simulink model "SendToUdpServer"  (R2018a)
settings: Solver=FixedStepAuto  StartTime=0.0  StopTime=inf  RelTol=1e-3  EnableMultiTasking=on
libraries: arduinowifilib x1
settings Model: SimulationMode=external  ExtModeTrigDuration=2  Creator=Gerard  LastModifiedBy=gaharkem
settings OptimizationCC: EnhancedBackFolding=on  PassReuseOutputArgsThreshold=0  MaxStackSize=64  OptimizeBlockOrder=speed  DifferentSizesBufferReuse=on  OptimizationCustomize=off
settings DebuggingCC: ParameterTunabilityLossMsg=error  LibraryContextMissingDiagnostic=warning
settings HardwareCC: ProdBitPerPointer=32  ProdBitPerSizeT=32  ProdBitPerPtrDiffT=32  ProdLargestAtomicInteger=Long  ProdLargestAtomicFloat=Double  ProdWordSize=32  ProdHWDeviceType=ARM Compatible->ARM Cortex  UseEmbeddedCoderFeatures=off  UseSimulinkCoderFeatures=off
settings SFSimCC: SimUseLocalCustomCode=on  MATLABDynamicMemAlloc=off
settings RTWCC: SystemTargetFile=ert.tlc  HardwareBoard=Arduino MKR1000  TLCOptions=-aInlineSetEventsForThisBaseRateFcn=TLC_FALSE -aSuppressMultiTaskScheduler=TLC_FALSE -aRateBasedStepFcn=1  TemplateMakefile=ert_default_tmf  GenerateReport=on  RTWUseLocalCustomCode=on  Toolchain=Arduino ARM  BuildConfiguration=Faster Runs  LaunchReport=on
settings CodeAppCC: ForceParamTrailComments=on  OperatorAnnotations=on
settings ERTTargetCC: ERTCustomFileBanners=off  SupportContinuousTime=on  SupportNonInlinedSFcns=on  RemoveResetFunc=off  SupportVariableSizeSignals=on  ModelStepFunctionPrototypeControlCompliant=off

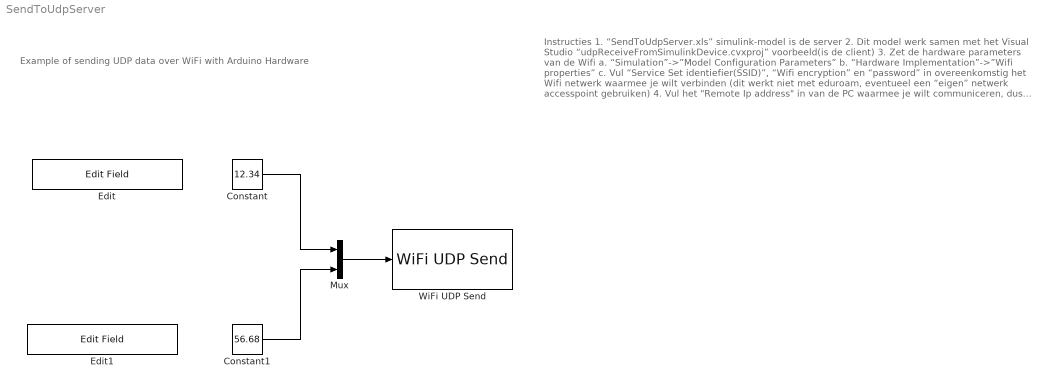
== system SendToUdpServer ==
  note: Example of sending UDP data over WiFi
      | with Arduino Hardware
  note: Instructies
      | 1. “SendToUdpServer.xls” simulink-model is de server
      | 2. Dit model werk samen met het Visual Studio “udpReceiveFromSimulinkDevice.cvxproj” voorbeeld(is de client)
      | 3. Zet de hardware parameters van de Wifi
      | a. “Simulation”->”Model Configuration Parameters”
      | b. “Hardware Implementation”->”Wifi properties”
      | c. Vul “Service Set identiefier(SSID)”, “Wifi encryption” en “password” in overeenkomstig het Wifi netwerk waarmee je wilt verbinden (dit werkt niet met eduroam, eventueel een “eigen” netwerk accesspoint gebruiken)
      | 4. Vul het "Remote Ip address" in van de PC waarmee je wilt communiceren, dus waar het visual Visula Studio programma " udpReceiveFromSimulinkDevice" op draait
      | 5. Start het “SendToUdpServer.xls” simulink-model
      | a. Als het model is gestart kun je zien wel ip-address er aan het model is toegewezen door het accesspoint, click het “View diagnostics” item onderaan het model(alleen zichtbaar al het model in running is)
      | 6. Vul het ip-address van de server in het bestand “tcpReceiveFromSimulinkDevice.cpp” in op de regel van “#define IP_ADDRESS "192.168.2.87"
      | 7. Start "tcpReceiveFromSimulinkDevice.cvxproj" Visual Studio project
      | Auteur: Gerard Harkema
      | Versie: 1.0
      | Datum: 6 april 2019
  Constant : Constant  Value=12.34  OutDataTypeStr=double
  Constant1 : Constant  Value=56.68  OutDataTypeStr=double
  Edit : EditField  WebBlockId=31  LabelPosition=Hide  Alignment=Center
  Edit1 : EditField  WebBlockId=32  LabelPosition=Hide  Alignment=Center
  Mux : Mux  Inputs=2
  WiFi UDP Send : arduinowifilib/WiFi UDP Send  remoteIPOctetString=192.168.2.74  remoteport=50002  localport=50001  remoteipoctet1=192  remoteipoctet2=168  remoteipoctet3=2  remoteipoctet4=74  wifiUDPIndex=0  blockPlatform=ARDUINO  isARMArch=true
      settings: SourceProductName=Simulink Support Package for Arduino Hardware  SourceProductBaseCode=ARDUINO
  wires:
  Constant/1 -> Mux/1
  Constant1/1 -> Mux/2
  Mux/1 -> WiFi UDP Send/1
